simulink model "Simulation"  (R2018b)
settings: Solver=VariableStepAuto  StartTime=0.0  StopTime=tmax  RelTol=1e-3
values from neighbouring files (symbols this model uses):
  BPden = [1 alpha]    [RunSimulation.m]
  BPnum = [0.3 alpha]    [RunSimulation.m]
  c = 250    [RunSimulation.m]
  Fb = -1*m    (= -90000)    [RunSimulation.m]
  l = 18    [RunSimulation.m]
  m = 90000    [RunSimulation.m]    (also in TractionCurve.m = 22500)
  p0 = 0    [RunSimulation.m]
  Pres = 0/1000*[5.7/771 0 1.6]    [RunSimulation.m]
  RBD = 5    [RunSimulation.m]
  tl = .1    (= 0.1)    [RunSimulation.m]
  v0 = 100/3.6    (= 27.7777777778)    [RunSimulation.m]
  VBD = 3.5    [RunSimulation.m]
(part 1 of 3)
settings Model: Creator=raphael  LastModifiedBy=raphael

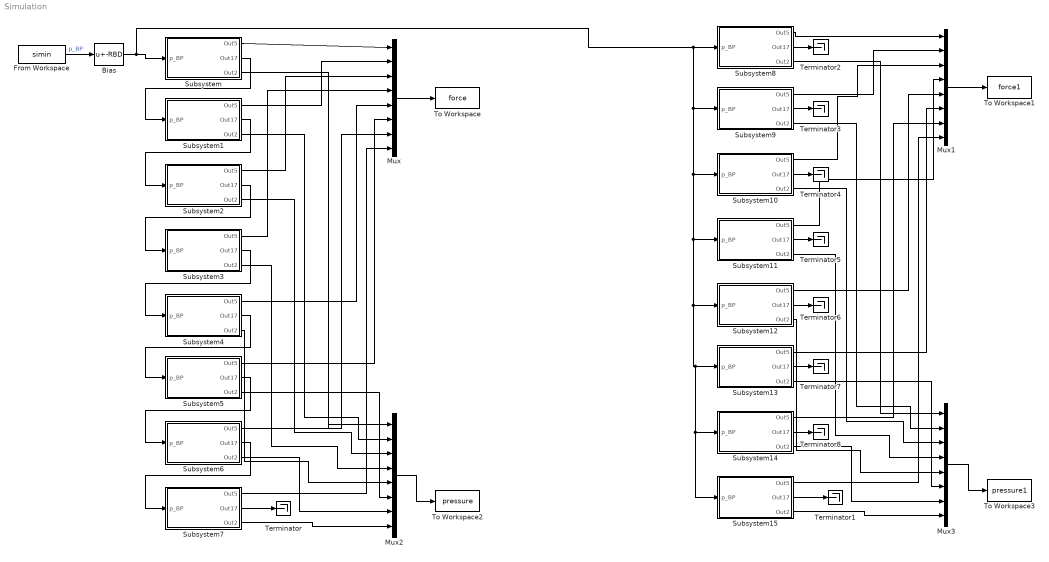
== system Simulation ==
  Bias : Bias  Bias=-RBD
  From Workspace : FromWorkspace  VariableName=simin  SampleTime=0
  Mux{,1..3} (4 alike) : Mux  Inputs=8
  Subsystem : Subsystem
  Subsystem1 : Subsystem
  Subsystem10 : Subsystem
  Subsystem11 : Subsystem
  Subsystem12 : Subsystem
  Subsystem13 : Subsystem
  Subsystem14 : Subsystem
  Subsystem15 : Subsystem
  Subsystem2 : Subsystem
  Subsystem3 : Subsystem
  Subsystem4 : Subsystem
  Subsystem5 : Subsystem
  Subsystem6 : Subsystem
  Subsystem7 : Subsystem
  Subsystem8 : Subsystem
  Subsystem9 : Subsystem
  Terminator{,1..8} (9 alike) : Terminator
  To Workspace : ToWorkspace  VariableName=force  SaveFormat=Timeseries  SampleTime=-1
  To Workspace1 : ToWorkspace  VariableName=force1  SaveFormat=Timeseries  SampleTime=-1
  To Workspace2 : ToWorkspace  VariableName=pressure  SaveFormat=Timeseries  SampleTime=-1
  To Workspace3 : ToWorkspace  VariableName=pressure1  SaveFormat=Timeseries  SampleTime=-1
  wires:
  Mux/1 -> To Workspace/1
  Mux2/1 -> To Workspace2/1
  From Workspace/1 -> Bias/1  "p_BP"
  Bias/1 -> Subsystem15/1(p_BP), Subsystem14/1(p_BP), Subsystem13/1(p_BP), Subsystem12/1(p_BP), Subsystem11/1(p_BP), Subsystem10/1(p_BP), Subsystem9/1(p_BP), Subsystem8/1(p_BP), Subsystem/1(p_BP)
  Subsystem/2(Out17) -> Subsystem1/1(p_BP)
  Subsystem1/2(Out17) -> Subsystem2/1(p_BP)
  Subsystem2/2(Out17) -> Subsystem3/1(p_BP)
  Subsystem3/2(Out17) -> Subsystem4/1(p_BP)
  Subsystem4/2(Out17) -> Subsystem5/1(p_BP)
  Subsystem5/2(Out17) -> Subsystem6/1(p_BP)
  Subsystem6/2(Out17) -> Subsystem7/1(p_BP)
  Subsystem7/2(Out17) -> Terminator/1
  Subsystem/1(Out5) -> Mux/1
  Subsystem1/1(Out5) -> Mux/2
  Subsystem2/1(Out5) -> Mux/3
  Subsystem3/1(Out5) -> Mux/4
  Subsystem4/1(Out5) -> Mux/5
  Subsystem5/1(Out5) -> Mux/6
  Subsystem6/1(Out5) -> Mux/7
  Subsystem7/1(Out5) -> Mux/8
  Subsystem1/3(Out2) -> Mux2/2
  Subsystem2/3(Out2) -> Mux2/3
  Subsystem3/3(Out2) -> Mux2/4
  Subsystem4/3(Out2) -> Mux2/5
  Subsystem/3(Out2) -> Mux2/1
  Subsystem5/3(Out2) -> Mux2/6
  Subsystem6/3(Out2) -> Mux2/7
  Subsystem7/3(Out2) -> Mux2/8
  Subsystem15/2(Out17) -> Terminator1/1
  Subsystem11/1(Out5) -> Mux1/4
  Subsystem8/3(Out2) -> Mux3/1
  Subsystem12/1(Out5) -> Mux1/5
  Subsystem8/1(Out5) -> Mux1/1
  Subsystem10/1(Out5) -> Mux1/3
  Subsystem9/3(Out2) -> Mux3/2
  Subsystem14/3(Out2) -> Mux3/7
  Subsystem14/1(Out5) -> Mux1/7
  Mux1/1 -> To Workspace1/1
  Subsystem10/3(Out2) -> Mux3/3
  Subsystem9/1(Out5) -> Mux1/2
  Subsystem12/3(Out2) -> Mux3/5
  Subsystem13/1(Out5) -> Mux1/6
  Mux3/1 -> To Workspace3/1
  Subsystem15/3(Out2) -> Mux3/8
  Subsystem13/3(Out2) -> Mux3/6
  Subsystem11/3(Out2) -> Mux3/4
  Subsystem15/1(Out5) -> Mux1/8
  Subsystem8/2(Out17) -> Terminator2/1
  Subsystem9/2(Out17) -> Terminator3/1
  Subsystem10/2(Out17) -> Terminator4/1
  Subsystem11/2(Out17) -> Terminator5/1
  Subsystem12/2(Out17) -> Terminator6/1
  Subsystem13/2(Out17) -> Terminator7/1
  Subsystem14/2(Out17) -> Terminator8/1

== system Simulation/Subsystem ==
  p_BP : Inport
  Mux : Mux  Inputs=5
  Mux2 : Mux  Inputs=5
  Wagon model : Subsystem
  Wagon model1 : Subsystem
  Wagon model2 : Subsystem
  Wagon model3 : Subsystem
  Wagon model4 : Subsystem
  Out5 : Outport
  Out17 : Outport  Port=2
  Out2 : Outport  Port=3
  wires:
  Wagon model3/2(p_BP_out) -> Mux2/4, Wagon model4/1(p_BP)
  Mux/1 -> Out5/1  "F_vec"
  Wagon model1/2(p_BP_out) -> Mux2/2, Wagon model2/1(p_BP)
  Wagon model4/2(p_BP_out) -> Out17/1, Mux2/5  "p_BP_out"
  Wagon model4/1(Fres) -> Mux/5
  Wagon model2/2(p_BP_out) -> Wagon model3/1(p_BP), Mux2/3
  Wagon model/2(p_BP_out) -> Mux2/1, Wagon model1/1(p_BP)
  Wagon model3/1(Fres) -> Mux/4
  Wagon model2/1(Fres) -> Mux/3
  Wagon model1/1(Fres) -> Mux/2
  Wagon model/1(Fres) -> Mux/1
  Mux2/1 -> Out2/1  "BP_vec"
  p_BP/1 -> Wagon model/1(p_BP)

== system Simulation/Subsystem1 ==
  p_BP : Inport
  Mux : Mux  Inputs=5
  Mux2 : Mux  Inputs=5
  Wagon model : Subsystem
  Wagon model1 : Subsystem
  Wagon model2 : Subsystem
  Wagon model3 : Subsystem
  Wagon model4 : Subsystem
  Out5 : Outport
  Out17 : Outport  Port=2
  Out2 : Outport  Port=3
  wires:
  Wagon model3/2(p_BP_out) -> Mux2/4, Wagon model4/1(p_BP)
  Mux/1 -> Out5/1  "F_vec"
  Wagon model1/2(p_BP_out) -> Mux2/2, Wagon model2/1(p_BP)
  Wagon model4/2(p_BP_out) -> Out17/1, Mux2/5  "p_BP_out"
  Wagon model4/1(Fres) -> Mux/5
  Wagon model2/2(p_BP_out) -> Wagon model3/1(p_BP), Mux2/3
  Wagon model/2(p_BP_out) -> Mux2/1, Wagon model1/1(p_BP)
  Wagon model3/1(Fres) -> Mux/4
  Wagon model2/1(Fres) -> Mux/3
  Wagon model1/1(Fres) -> Mux/2
  Wagon model/1(Fres) -> Mux/1
  Mux2/1 -> Out2/1  "BP_vec"
  p_BP/1 -> Wagon model/1(p_BP)

== system Simulation/Subsystem10 ==
  p_BP : Inport
  Mux : Mux  Inputs=5
  Mux2 : Mux  Inputs=5
  Wagon model : Subsystem
  Wagon model1 : Subsystem
  Wagon model2 : Subsystem
  Wagon model3 : Subsystem
  Wagon model4 : Subsystem
  Out5 : Outport
  Out17 : Outport  Port=2
  Out2 : Outport  Port=3
  wires:
  Wagon model3/2(p_BP_out) -> Mux2/4, Wagon model4/1(p_BP)
  Mux/1 -> Out5/1  "F_vec"
  Wagon model1/2(p_BP_out) -> Mux2/2, Wagon model2/1(p_BP)
  Wagon model4/2(p_BP_out) -> Out17/1, Mux2/5  "p_BP_out"
  Wagon model4/1(Fres) -> Mux/5
  Wagon model2/2(p_BP_out) -> Wagon model3/1(p_BP), Mux2/3
  Wagon model/2(p_BP_out) -> Mux2/1, Wagon model1/1(p_BP)
  Wagon model3/1(Fres) -> Mux/4
  Wagon model2/1(Fres) -> Mux/3
  Wagon model1/1(Fres) -> Mux/2
  Wagon model/1(Fres) -> Mux/1
  Mux2/1 -> Out2/1  "BP_vec"
  p_BP/1 -> Wagon model/1(p_BP)

== system Simulation/Subsystem11 ==
  p_BP : Inport
  Mux : Mux  Inputs=5
  Mux2 : Mux  Inputs=5
  Wagon model : Subsystem
  Wagon model1 : Subsystem
  Wagon model2 : Subsystem
  Wagon model3 : Subsystem
  Wagon model4 : Subsystem
  Out5 : Outport
  Out17 : Outport  Port=2
  Out2 : Outport  Port=3
  wires:
  Wagon model3/2(p_BP_out) -> Mux2/4, Wagon model4/1(p_BP)
  Mux/1 -> Out5/1  "F_vec"
  Wagon model1/2(p_BP_out) -> Mux2/2, Wagon model2/1(p_BP)
  Wagon model4/2(p_BP_out) -> Out17/1, Mux2/5  "p_BP_out"
  Wagon model4/1(Fres) -> Mux/5
  Wagon model2/2(p_BP_out) -> Wagon model3/1(p_BP), Mux2/3
  Wagon model/2(p_BP_out) -> Mux2/1, Wagon model1/1(p_BP)
  Wagon model3/1(Fres) -> Mux/4
  Wagon model2/1(Fres) -> Mux/3
  Wagon model1/1(Fres) -> Mux/2
  Wagon model/1(Fres) -> Mux/1
  Mux2/1 -> Out2/1  "BP_vec"
  p_BP/1 -> Wagon model/1(p_BP)

== system Simulation/Subsystem12 ==
  p_BP : Inport
  Mux : Mux  Inputs=5
  Mux2 : Mux  Inputs=5
  Wagon model : Subsystem
  Wagon model1 : Subsystem
  Wagon model2 : Subsystem
  Wagon model3 : Subsystem
  Wagon model4 : Subsystem
  Out5 : Outport
  Out17 : Outport  Port=2
  Out2 : Outport  Port=3
  wires:
  Wagon model3/2(p_BP_out) -> Mux2/4, Wagon model4/1(p_BP)
  Mux/1 -> Out5/1  "F_vec"
  Wagon model1/2(p_BP_out) -> Mux2/2, Wagon model2/1(p_BP)
  Wagon model4/2(p_BP_out) -> Out17/1, Mux2/5  "p_BP_out"
  Wagon model4/1(Fres) -> Mux/5
  Wagon model2/2(p_BP_out) -> Wagon model3/1(p_BP), Mux2/3
  Wagon model/2(p_BP_out) -> Mux2/1, Wagon model1/1(p_BP)
  Wagon model3/1(Fres) -> Mux/4
  Wagon model2/1(Fres) -> Mux/3
  Wagon model1/1(Fres) -> Mux/2
  Wagon model/1(Fres) -> Mux/1
  Mux2/1 -> Out2/1  "BP_vec"
  p_BP/1 -> Wagon model/1(p_BP)

== system Simulation/Subsystem13 ==
  p_BP : Inport
  Mux : Mux  Inputs=5
  Mux2 : Mux  Inputs=5
  Wagon model : Subsystem
  Wagon model1 : Subsystem
  Wagon model2 : Subsystem
  Wagon model3 : Subsystem
  Wagon model4 : Subsystem
  Out5 : Outport
  Out17 : Outport  Port=2
  Out2 : Outport  Port=3
  wires:
  Wagon model3/2(p_BP_out) -> Mux2/4, Wagon model4/1(p_BP)
  Mux/1 -> Out5/1  "F_vec"
  Wagon model1/2(p_BP_out) -> Mux2/2, Wagon model2/1(p_BP)
  Wagon model4/2(p_BP_out) -> Out17/1, Mux2/5  "p_BP_out"
  Wagon model4/1(Fres) -> Mux/5
  Wagon model2/2(p_BP_out) -> Wagon model3/1(p_BP), Mux2/3
  Wagon model/2(p_BP_out) -> Mux2/1, Wagon model1/1(p_BP)
  Wagon model3/1(Fres) -> Mux/4
  Wagon model2/1(Fres) -> Mux/3
  Wagon model1/1(Fres) -> Mux/2
  Wagon model/1(Fres) -> Mux/1
  Mux2/1 -> Out2/1  "BP_vec"
  p_BP/1 -> Wagon model/1(p_BP)

== system Simulation/Subsystem14 ==
  p_BP : Inport
  Mux : Mux  Inputs=5
  Mux2 : Mux  Inputs=5
  Wagon model : Subsystem
  Wagon model1 : Subsystem
  Wagon model2 : Subsystem
  Wagon model3 : Subsystem
  Wagon model4 : Subsystem
  Out5 : Outport
  Out17 : Outport  Port=2
  Out2 : Outport  Port=3
  wires:
  Wagon model3/2(p_BP_out) -> Mux2/4, Wagon model4/1(p_BP)
  Mux/1 -> Out5/1  "F_vec"
  Wagon model1/2(p_BP_out) -> Mux2/2, Wagon model2/1(p_BP)
  Wagon model4/2(p_BP_out) -> Out17/1, Mux2/5  "p_BP_out"
  Wagon model4/1(Fres) -> Mux/5
  Wagon model2/2(p_BP_out) -> Wagon model3/1(p_BP), Mux2/3
  Wagon model/2(p_BP_out) -> Mux2/1, Wagon model1/1(p_BP)
  Wagon model3/1(Fres) -> Mux/4
  Wagon model2/1(Fres) -> Mux/3
  Wagon model1/1(Fres) -> Mux/2
  Wagon model/1(Fres) -> Mux/1
  Mux2/1 -> Out2/1  "BP_vec"
  p_BP/1 -> Wagon model/1(p_BP)

== system Simulation/Subsystem15 ==
  p_BP : Inport
  Mux : Mux  Inputs=5
  Mux2 : Mux  Inputs=5
  Wagon model : Subsystem
  Wagon model1 : Subsystem
  Wagon model2 : Subsystem
  Wagon model3 : Subsystem
  Wagon model4 : Subsystem
  Out5 : Outport
  Out17 : Outport  Port=2
  Out2 : Outport  Port=3
  wires:
  Wagon model3/2(p_BP_out) -> Mux2/4, Wagon model4/1(p_BP)
  Mux/1 -> Out5/1  "F_vec"
  Wagon model1/2(p_BP_out) -> Mux2/2, Wagon model2/1(p_BP)
  Wagon model4/2(p_BP_out) -> Out17/1, Mux2/5  "p_BP_out"
  Wagon model4/1(Fres) -> Mux/5
  Wagon model2/2(p_BP_out) -> Wagon model3/1(p_BP), Mux2/3
  Wagon model/2(p_BP_out) -> Mux2/1, Wagon model1/1(p_BP)
  Wagon model3/1(Fres) -> Mux/4
  Wagon model2/1(Fres) -> Mux/3
  Wagon model1/1(Fres) -> Mux/2
  Wagon model/1(Fres) -> Mux/1
  Mux2/1 -> Out2/1  "BP_vec"
  p_BP/1 -> Wagon model/1(p_BP)

== system Simulation/Subsystem2 ==
  p_BP : Inport
  Mux : Mux  Inputs=5
  Mux2 : Mux  Inputs=5
  Wagon model : Subsystem
  Wagon model1 : Subsystem
  Wagon model2 : Subsystem
  Wagon model3 : Subsystem
  Wagon model4 : Subsystem
  Out5 : Outport
  Out17 : Outport  Port=2
  Out2 : Outport  Port=3
  wires:
  Wagon model3/2(p_BP_out) -> Mux2/4, Wagon model4/1(p_BP)
  Mux/1 -> Out5/1  "F_vec"
  Wagon model1/2(p_BP_out) -> Mux2/2, Wagon model2/1(p_BP)
  Wagon model4/2(p_BP_out) -> Out17/1, Mux2/5  "p_BP_out"
  Wagon model4/1(Fres) -> Mux/5
  Wagon model2/2(p_BP_out) -> Wagon model3/1(p_BP), Mux2/3
  Wagon model/2(p_BP_out) -> Mux2/1, Wagon model1/1(p_BP)
  Wagon model3/1(Fres) -> Mux/4
  Wagon model2/1(Fres) -> Mux/3
  Wagon model1/1(Fres) -> Mux/2
  Wagon model/1(Fres) -> Mux/1
  Mux2/1 -> Out2/1  "BP_vec"
  p_BP/1 -> Wagon model/1(p_BP)

== system Simulation/Subsystem3 ==
  p_BP : Inport
  Mux : Mux  Inputs=5
  Mux2 : Mux  Inputs=5
  Wagon model : Subsystem
  Wagon model1 : Subsystem
  Wagon model2 : Subsystem
  Wagon model3 : Subsystem
  Wagon model4 : Subsystem
  Out5 : Outport
  Out17 : Outport  Port=2
  Out2 : Outport  Port=3
  wires:
  Wagon model3/2(p_BP_out) -> Mux2/4, Wagon model4/1(p_BP)
  Mux/1 -> Out5/1  "F_vec"
  Wagon model1/2(p_BP_out) -> Mux2/2, Wagon model2/1(p_BP)
  Wagon model4/2(p_BP_out) -> Out17/1, Mux2/5  "p_BP_out"
  Wagon model4/1(Fres) -> Mux/5
  Wagon model2/2(p_BP_out) -> Wagon model3/1(p_BP), Mux2/3
  Wagon model/2(p_BP_out) -> Mux2/1, Wagon model1/1(p_BP)
  Wagon model3/1(Fres) -> Mux/4
  Wagon model2/1(Fres) -> Mux/3
  Wagon model1/1(Fres) -> Mux/2
  Wagon model/1(Fres) -> Mux/1
  Mux2/1 -> Out2/1  "BP_vec"
  p_BP/1 -> Wagon model/1(p_BP)

== system Simulation/Subsystem4 ==
  p_BP : Inport
  Mux : Mux  Inputs=5
  Mux2 : Mux  Inputs=5
  Wagon model : Subsystem
  Wagon model1 : Subsystem
  Wagon model2 : Subsystem
  Wagon model3 : Subsystem
  Wagon model4 : Subsystem
  Out5 : Outport
  Out17 : Outport  Port=2
  Out2 : Outport  Port=3
  wires:
  Wagon model3/2(p_BP_out) -> Mux2/4, Wagon model4/1(p_BP)
  Mux/1 -> Out5/1  "F_vec"
  Wagon model1/2(p_BP_out) -> Mux2/2, Wagon model2/1(p_BP)
  Wagon model4/2(p_BP_out) -> Out17/1, Mux2/5  "p_BP_out"
  Wagon model4/1(Fres) -> Mux/5
  Wagon model2/2(p_BP_out) -> Wagon model3/1(p_BP), Mux2/3
  Wagon model/2(p_BP_out) -> Mux2/1, Wagon model1/1(p_BP)
  Wagon model3/1(Fres) -> Mux/4
  Wagon model2/1(Fres) -> Mux/3
  Wagon model1/1(Fres) -> Mux/2
  Wagon model/1(Fres) -> Mux/1
  Mux2/1 -> Out2/1  "BP_vec"
  p_BP/1 -> Wagon model/1(p_BP)

== system Simulation/Subsystem5 ==
  p_BP : Inport
  Mux : Mux  Inputs=5
  Mux2 : Mux  Inputs=5
  Wagon model : Subsystem
  Wagon model1 : Subsystem
  Wagon model2 : Subsystem
  Wagon model3 : Subsystem
  Wagon model4 : Subsystem
  Out5 : Outport
  Out17 : Outport  Port=2
  Out2 : Outport  Port=3
  wires:
  Wagon model3/2(p_BP_out) -> Mux2/4, Wagon model4/1(p_BP)
  Mux/1 -> Out5/1  "F_vec"
  Wagon model1/2(p_BP_out) -> Mux2/2, Wagon model2/1(p_BP)
  Wagon model4/2(p_BP_out) -> Out17/1, Mux2/5  "p_BP_out"
  Wagon model4/1(Fres) -> Mux/5
  Wagon model2/2(p_BP_out) -> Wagon model3/1(p_BP), Mux2/3
  Wagon model/2(p_BP_out) -> Mux2/1, Wagon model1/1(p_BP)
  Wagon model3/1(Fres) -> Mux/4
  Wagon model2/1(Fres) -> Mux/3
  Wagon model1/1(Fres) -> Mux/2
  Wagon model/1(Fres) -> Mux/1
  Mux2/1 -> Out2/1  "BP_vec"
  p_BP/1 -> Wagon model/1(p_BP)

== system Simulation/Subsystem6 ==
  p_BP : Inport
  Mux : Mux  Inputs=5
  Mux2 : Mux  Inputs=5
  Wagon model : Subsystem
  Wagon model1 : Subsystem
  Wagon model2 : Subsystem
  Wagon model3 : Subsystem
  Wagon model4 : Subsystem
  Out5 : Outport
  Out17 : Outport  Port=2
  Out2 : Outport  Port=3
  wires:
  Wagon model3/2(p_BP_out) -> Mux2/4, Wagon model4/1(p_BP)
  Mux/1 -> Out5/1  "F_vec"
  Wagon model1/2(p_BP_out) -> Mux2/2, Wagon model2/1(p_BP)
  Wagon model4/2(p_BP_out) -> Out17/1, Mux2/5  "p_BP_out"
  Wagon model4/1(Fres) -> Mux/5
  Wagon model2/2(p_BP_out) -> Wagon model3/1(p_BP), Mux2/3
  Wagon model/2(p_BP_out) -> Mux2/1, Wagon model1/1(p_BP)
  Wagon model3/1(Fres) -> Mux/4
  Wagon model2/1(Fres) -> Mux/3
  Wagon model1/1(Fres) -> Mux/2
  Wagon model/1(Fres) -> Mux/1
  Mux2/1 -> Out2/1  "BP_vec"
  p_BP/1 -> Wagon model/1(p_BP)

== system Simulation/Subsystem7 ==
  p_BP : Inport
  Mux : Mux  Inputs=5
  Mux2 : Mux  Inputs=5
  Wagon model : Subsystem
  Wagon model1 : Subsystem
  Wagon model2 : Subsystem
  Wagon model3 : Subsystem
  Wagon model4 : Subsystem
  Out5 : Outport
  Out17 : Outport  Port=2
  Out2 : Outport  Port=3
  wires:
  Wagon model3/2(p_BP_out) -> Mux2/4, Wagon model4/1(p_BP)
  Mux/1 -> Out5/1  "F_vec"
  Wagon model1/2(p_BP_out) -> Mux2/2, Wagon model2/1(p_BP)
  Wagon model4/2(p_BP_out) -> Out17/1, Mux2/5  "p_BP_out"
  Wagon model4/1(Fres) -> Mux/5
  Wagon model2/2(p_BP_out) -> Wagon model3/1(p_BP), Mux2/3
  Wagon model/2(p_BP_out) -> Mux2/1, Wagon model1/1(p_BP)
  Wagon model3/1(Fres) -> Mux/4
  Wagon model2/1(Fres) -> Mux/3
  Wagon model1/1(Fres) -> Mux/2
  Wagon model/1(Fres) -> Mux/1
  Mux2/1 -> Out2/1  "BP_vec"
  p_BP/1 -> Wagon model/1(p_BP)

== system Simulation/Subsystem8 ==
  p_BP : Inport
  Mux : Mux  Inputs=5
  Mux2 : Mux  Inputs=5
  Wagon model : Subsystem
  Wagon model1 : Subsystem
  Wagon model2 : Subsystem
  Wagon model3 : Subsystem
  Wagon model4 : Subsystem
  Out5 : Outport
  Out17 : Outport  Port=2
  Out2 : Outport  Port=3
  wires:
  Wagon model3/2(p_BP_out) -> Mux2/4, Wagon model4/1(p_BP)
  Mux/1 -> Out5/1  "F_vec"
  Wagon model1/2(p_BP_out) -> Mux2/2, Wagon model2/1(p_BP)
  Wagon model4/2(p_BP_out) -> Out17/1, Mux2/5  "p_BP_out"
  Wagon model4/1(Fres) -> Mux/5
  Wagon model2/2(p_BP_out) -> Wagon model3/1(p_BP), Mux2/3
  Wagon model/2(p_BP_out) -> Mux2/1, Wagon model1/1(p_BP)
  Wagon model3/1(Fres) -> Mux/4
  Wagon model2/1(Fres) -> Mux/3
  Wagon model1/1(Fres) -> Mux/2
  Wagon model/1(Fres) -> Mux/1
  Mux2/1 -> Out2/1  "BP_vec"
  p_BP/1 -> Wagon model/1(p_BP)

== system Simulation/Subsystem9 ==
  p_BP : Inport
  Mux : Mux  Inputs=5
  Mux2 : Mux  Inputs=5
  Wagon model : Subsystem
  Wagon model1 : Subsystem
  Wagon model2 : Subsystem
  Wagon model3 : Subsystem
  Wagon model4 : Subsystem
  Out5 : Outport
  Out17 : Outport  Port=2
  Out2 : Outport  Port=3
  wires:
  Wagon model3/2(p_BP_out) -> Mux2/4, Wagon model4/1(p_BP)
  Mux/1 -> Out5/1  "F_vec"
  Wagon model1/2(p_BP_out) -> Mux2/2, Wagon model2/1(p_BP)
  Wagon model4/2(p_BP_out) -> Out17/1, Mux2/5  "p_BP_out"
  Wagon model4/1(Fres) -> Mux/5
  Wagon model2/2(p_BP_out) -> Wagon model3/1(p_BP), Mux2/3
  Wagon model/2(p_BP_out) -> Mux2/1, Wagon model1/1(p_BP)
  Wagon model3/1(Fres) -> Mux/4
  Wagon model2/1(Fres) -> Mux/3
  Wagon model1/1(Fres) -> Mux/2
  Wagon model/1(Fres) -> Mux/1
  Mux2/1 -> Out2/1  "BP_vec"
  p_BP/1 -> Wagon model/1(p_BP)

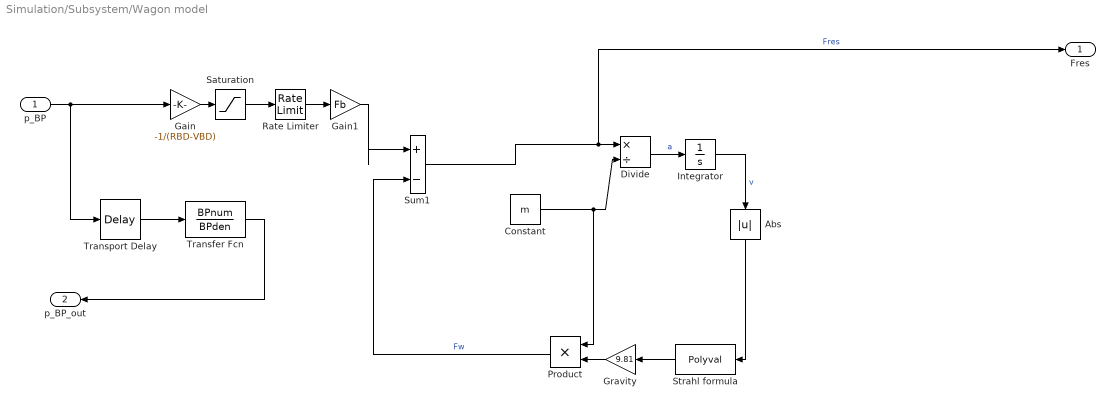
== system Simulation/Subsystem/Wagon model ==
  p_BP : Inport
  Abs : Abs
  Constant : Constant  Value=m
  Divide : Product  Inputs=*/
  Gain : Gain  Gain=-1/(RBD-VBD)
  Gain1 : Gain  Gain=Fb
  Gravity : Gain  Gain=9.81
  Integrator : Integrator  InitialCondition=v0
  Product : Product
  Rate Limiter : RateLimiter  RisingSlewLimit=1/tf  FallingSlewLimit=-1/tl  SampleTimeMode=inherited
  Saturation : Saturate  UpperLimit=1  LowerLimit=0
  Strahl formula : Polyval  Coefs=Pres
  Sum1 : Sum  Inputs=|+-
  Transfer Fcn : TransferFcn  Numerator=BPnum  Denominator=BPden
  Transport Delay : TransportDelay  DelayTime=l/c  InitialOutput=p0
  Fres : Outport
  p_BP_out : Outport  Port=2
  wires:
  Sum1/1 -> Fres/1, Divide/1  "Fres"
  Strahl formula/1 -> Gravity/1
  Abs/1 -> Strahl formula/1
  Gravity/1 -> Product/2
  Product/1 -> Sum1/2  "Fw"
  Integrator/1 -> Abs/1  "v"
  Constant/1 -> Product/1, Divide/2
  Divide/1 -> Integrator/1  "a"
  p_BP/1 -> Gain/1, Transport Delay/1
  Gain/1 -> Saturation/1
  Gain1/1 -> Sum1/1
  Saturation/1 -> Rate Limiter/1
  Rate Limiter/1 -> Gain1/1
  Transfer Fcn/1 -> p_BP_out/1
  Transport Delay/1 -> Transfer Fcn/1

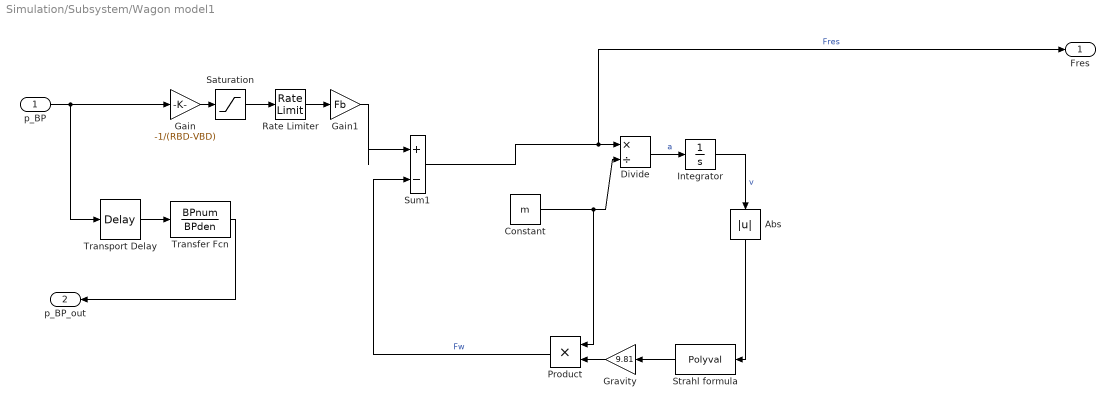
== system Simulation/Subsystem/Wagon model1 ==
  p_BP : Inport
  Abs : Abs
  Constant : Constant  Value=m
  Divide : Product  Inputs=*/
  Gain : Gain  Gain=-1/(RBD-VBD)
  Gain1 : Gain  Gain=Fb
  Gravity : Gain  Gain=9.81
  Integrator : Integrator  InitialCondition=v0
  Product : Product
  Rate Limiter : RateLimiter  RisingSlewLimit=1/tf  FallingSlewLimit=-1/tl  SampleTimeMode=inherited
  Saturation : Saturate  UpperLimit=1  LowerLimit=0
  Strahl formula : Polyval  Coefs=Pres
  Sum1 : Sum  Inputs=|+-
  Transfer Fcn : TransferFcn  Numerator=BPnum  Denominator=BPden
  Transport Delay : TransportDelay  DelayTime=l/c  InitialOutput=p0
  Fres : Outport
  p_BP_out : Outport  Port=2
  wires:
  Sum1/1 -> Fres/1, Divide/1  "Fres"
  Strahl formula/1 -> Gravity/1
  Abs/1 -> Strahl formula/1
  Gravity/1 -> Product/2
  Product/1 -> Sum1/2  "Fw"
  Integrator/1 -> Abs/1  "v"
  Constant/1 -> Product/1, Divide/2
  Divide/1 -> Integrator/1  "a"
  p_BP/1 -> Gain/1, Transport Delay/1
  Gain/1 -> Saturation/1
  Gain1/1 -> Sum1/1
  Saturation/1 -> Rate Limiter/1
  Rate Limiter/1 -> Gain1/1
  Transport Delay/1 -> Transfer Fcn/1
  Transfer Fcn/1 -> p_BP_out/1

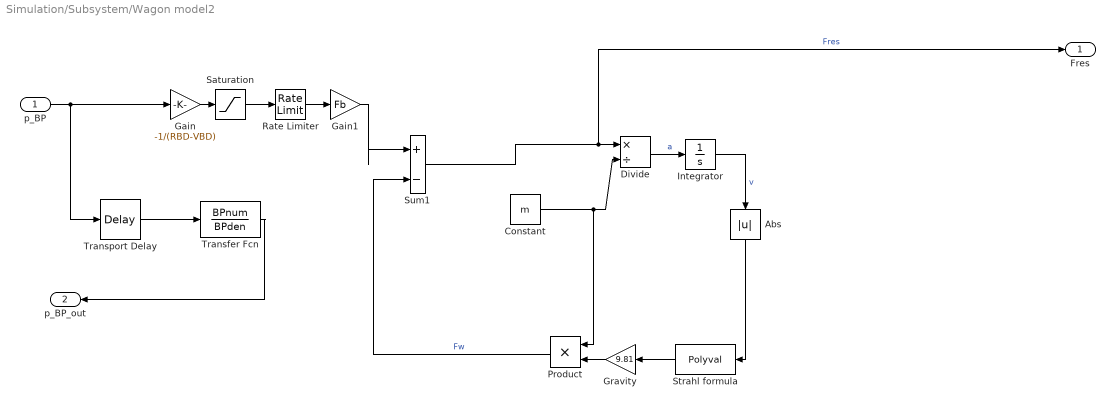
== system Simulation/Subsystem/Wagon model2 ==
  p_BP : Inport
  Abs : Abs
  Constant : Constant  Value=m
  Divide : Product  Inputs=*/
  Gain : Gain  Gain=-1/(RBD-VBD)
  Gain1 : Gain  Gain=Fb
  Gravity : Gain  Gain=9.81
  Integrator : Integrator  InitialCondition=v0
  Product : Product
  Rate Limiter : RateLimiter  RisingSlewLimit=1/tf  FallingSlewLimit=-1/tl  SampleTimeMode=inherited
  Saturation : Saturate  UpperLimit=1  LowerLimit=0
  Strahl formula : Polyval  Coefs=Pres
  Sum1 : Sum  Inputs=|+-
  Transfer Fcn : TransferFcn  Numerator=BPnum  Denominator=BPden
  Transport Delay : TransportDelay  DelayTime=l/c  InitialOutput=p0
  Fres : Outport
  p_BP_out : Outport  Port=2
  wires:
  Sum1/1 -> Fres/1, Divide/1  "Fres"
  Strahl formula/1 -> Gravity/1
  Abs/1 -> Strahl formula/1
  Gravity/1 -> Product/2
  Product/1 -> Sum1/2  "Fw"
  Constant/1 -> Product/1, Divide/2
  Divide/1 -> Integrator/1  "a"
  p_BP/1 -> Gain/1, Transport Delay/1
  Gain/1 -> Saturation/1
  Gain1/1 -> Sum1/1
  Saturation/1 -> Rate Limiter/1
  Rate Limiter/1 -> Gain1/1
  Transport Delay/1 -> Transfer Fcn/1
  Transfer Fcn/1 -> p_BP_out/1
  Integrator/1 -> Abs/1  "v"

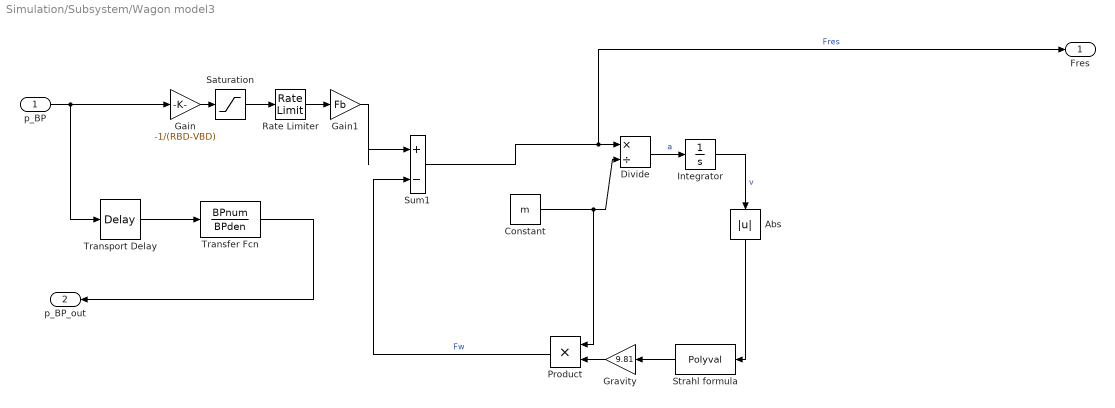
== system Simulation/Subsystem/Wagon model3 ==
  p_BP : Inport
  Abs : Abs
  Constant : Constant  Value=m
  Divide : Product  Inputs=*/
  Gain : Gain  Gain=-1/(RBD-VBD)
  Gain1 : Gain  Gain=Fb
  Gravity : Gain  Gain=9.81
  Integrator : Integrator  InitialCondition=v0
  Product : Product
  Rate Limiter : RateLimiter  RisingSlewLimit=1/tf  FallingSlewLimit=-1/tl  SampleTimeMode=inherited
  Saturation : Saturate  UpperLimit=1  LowerLimit=0
  Strahl formula : Polyval  Coefs=Pres
  Sum1 : Sum  Inputs=|+-
  Transfer Fcn : TransferFcn  Numerator=BPnum  Denominator=BPden
  Transport Delay : TransportDelay  DelayTime=l/c  InitialOutput=p0
  Fres : Outport
  p_BP_out : Outport  Port=2
  wires:
  Sum1/1 -> Fres/1, Divide/1  "Fres"
  Strahl formula/1 -> Gravity/1
  Abs/1 -> Strahl formula/1
  Gravity/1 -> Product/2
  Product/1 -> Sum1/2  "Fw"
  Constant/1 -> Product/1, Divide/2
  Divide/1 -> Integrator/1  "a"
  p_BP/1 -> Gain/1, Transport Delay/1
  Gain/1 -> Saturation/1
  Gain1/1 -> Sum1/1
  Saturation/1 -> Rate Limiter/1
  Rate Limiter/1 -> Gain1/1
  Transport Delay/1 -> Transfer Fcn/1
  Transfer Fcn/1 -> p_BP_out/1
  Integrator/1 -> Abs/1  "v"

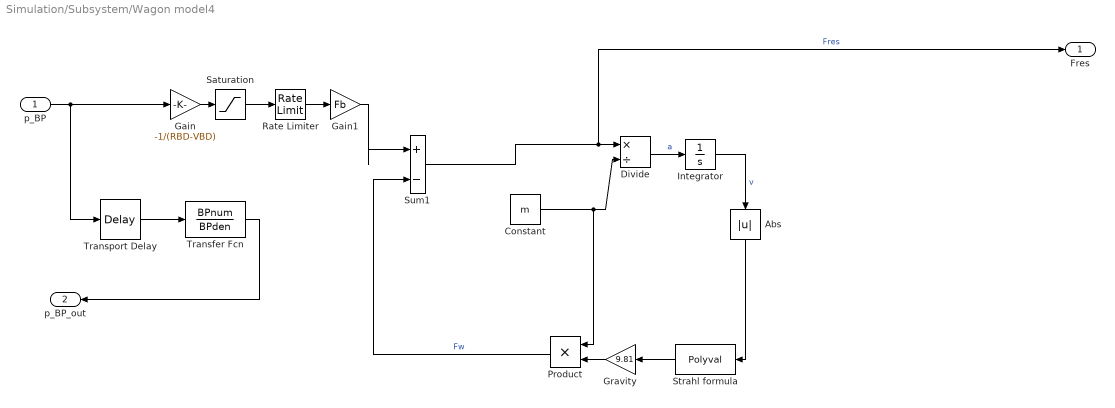
== system Simulation/Subsystem/Wagon model4 ==
  p_BP : Inport
  Abs : Abs
  Constant : Constant  Value=m
  Divide : Product  Inputs=*/
  Gain : Gain  Gain=-1/(RBD-VBD)
  Gain1 : Gain  Gain=Fb
  Gravity : Gain  Gain=9.81
  Integrator : Integrator  InitialCondition=v0
  Product : Product
  Rate Limiter : RateLimiter  RisingSlewLimit=1/tf  FallingSlewLimit=-1/tl  SampleTimeMode=inherited
  Saturation : Saturate  UpperLimit=1  LowerLimit=0
  Strahl formula : Polyval  Coefs=Pres
  Sum1 : Sum  Inputs=|+-
  Transfer Fcn : TransferFcn  Numerator=BPnum  Denominator=BPden
  Transport Delay : TransportDelay  DelayTime=l/c  InitialOutput=p0
  Fres : Outport
  p_BP_out : Outport  Port=2
  wires:
  Sum1/1 -> Fres/1, Divide/1  "Fres"
  Strahl formula/1 -> Gravity/1
  Abs/1 -> Strahl formula/1
  Gravity/1 -> Product/2
  Product/1 -> Sum1/2  "Fw"
  Integrator/1 -> Abs/1  "v"
  Constant/1 -> Product/1, Divide/2
  Divide/1 -> Integrator/1  "a"
  p_BP/1 -> Gain/1, Transport Delay/1
  Gain/1 -> Saturation/1
  Gain1/1 -> Sum1/1
  Saturation/1 -> Rate Limiter/1
  Rate Limiter/1 -> Gain1/1
  Transfer Fcn/1 -> p_BP_out/1
  Transport Delay/1 -> Transfer Fcn/1

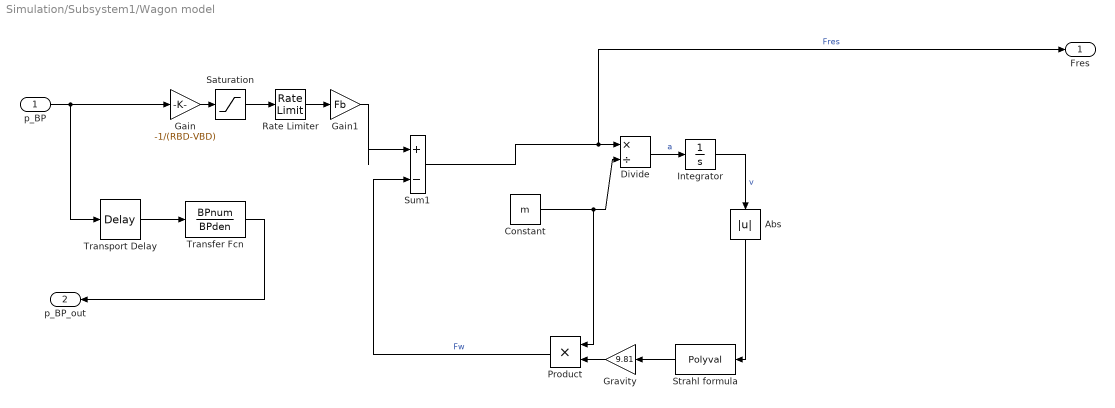
== system Simulation/Subsystem1/Wagon model ==
  p_BP : Inport
  Abs : Abs
  Constant : Constant  Value=m
  Divide : Product  Inputs=*/
  Gain : Gain  Gain=-1/(RBD-VBD)
  Gain1 : Gain  Gain=Fb
  Gravity : Gain  Gain=9.81
  Integrator : Integrator  InitialCondition=v0
  Product : Product
  Rate Limiter : RateLimiter  RisingSlewLimit=1/tf  FallingSlewLimit=-1/tl  SampleTimeMode=inherited
  Saturation : Saturate  UpperLimit=1  LowerLimit=0
  Strahl formula : Polyval  Coefs=Pres
  Sum1 : Sum  Inputs=|+-
  Transfer Fcn : TransferFcn  Numerator=BPnum  Denominator=BPden
  Transport Delay : TransportDelay  DelayTime=l/c  InitialOutput=p0
  Fres : Outport
  p_BP_out : Outport  Port=2
  wires:
  Sum1/1 -> Fres/1, Divide/1  "Fres"
  Strahl formula/1 -> Gravity/1
  Abs/1 -> Strahl formula/1
  Gravity/1 -> Product/2
  Product/1 -> Sum1/2  "Fw"
  Integrator/1 -> Abs/1  "v"
  Constant/1 -> Product/1, Divide/2
  Divide/1 -> Integrator/1  "a"
  p_BP/1 -> Gain/1, Transport Delay/1
  Gain/1 -> Saturation/1
  Gain1/1 -> Sum1/1
  Saturation/1 -> Rate Limiter/1
  Rate Limiter/1 -> Gain1/1
  Transfer Fcn/1 -> p_BP_out/1
  Transport Delay/1 -> Transfer Fcn/1

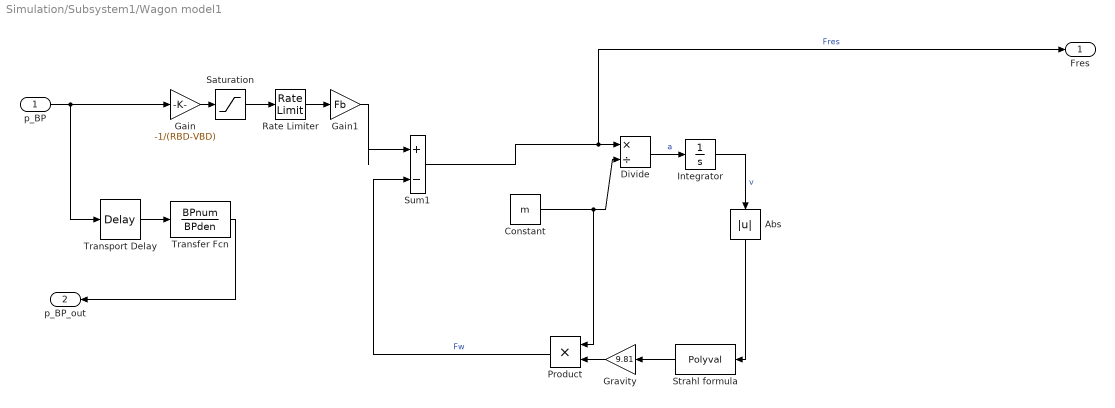
== system Simulation/Subsystem1/Wagon model1 ==
  p_BP : Inport
  Abs : Abs
  Constant : Constant  Value=m
  Divide : Product  Inputs=*/
  Gain : Gain  Gain=-1/(RBD-VBD)
  Gain1 : Gain  Gain=Fb
  Gravity : Gain  Gain=9.81
  Integrator : Integrator  InitialCondition=v0
  Product : Product
  Rate Limiter : RateLimiter  RisingSlewLimit=1/tf  FallingSlewLimit=-1/tl  SampleTimeMode=inherited
  Saturation : Saturate  UpperLimit=1  LowerLimit=0
  Strahl formula : Polyval  Coefs=Pres
  Sum1 : Sum  Inputs=|+-
  Transfer Fcn : TransferFcn  Numerator=BPnum  Denominator=BPden
  Transport Delay : TransportDelay  DelayTime=l/c  InitialOutput=p0
  Fres : Outport
  p_BP_out : Outport  Port=2
  wires:
  Sum1/1 -> Fres/1, Divide/1  "Fres"
  Strahl formula/1 -> Gravity/1
  Abs/1 -> Strahl formula/1
  Gravity/1 -> Product/2
  Product/1 -> Sum1/2  "Fw"
  Integrator/1 -> Abs/1  "v"
  Constant/1 -> Product/1, Divide/2
  Divide/1 -> Integrator/1  "a"
  p_BP/1 -> Gain/1, Transport Delay/1
  Gain/1 -> Saturation/1
  Gain1/1 -> Sum1/1
  Saturation/1 -> Rate Limiter/1
  Rate Limiter/1 -> Gain1/1
  Transport Delay/1 -> Transfer Fcn/1
  Transfer Fcn/1 -> p_BP_out/1

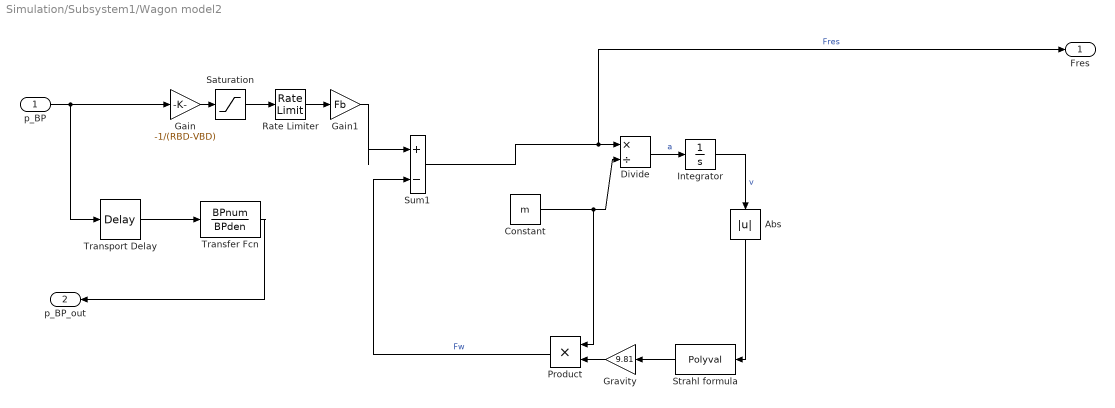
== system Simulation/Subsystem1/Wagon model2 ==
  p_BP : Inport
  Abs : Abs
  Constant : Constant  Value=m
  Divide : Product  Inputs=*/
  Gain : Gain  Gain=-1/(RBD-VBD)
  Gain1 : Gain  Gain=Fb
  Gravity : Gain  Gain=9.81
  Integrator : Integrator  InitialCondition=v0
  Product : Product
  Rate Limiter : RateLimiter  RisingSlewLimit=1/tf  FallingSlewLimit=-1/tl  SampleTimeMode=inherited
  Saturation : Saturate  UpperLimit=1  LowerLimit=0
  Strahl formula : Polyval  Coefs=Pres
  Sum1 : Sum  Inputs=|+-
  Transfer Fcn : TransferFcn  Numerator=BPnum  Denominator=BPden
  Transport Delay : TransportDelay  DelayTime=l/c  InitialOutput=p0
  Fres : Outport
  p_BP_out : Outport  Port=2
  wires:
  Sum1/1 -> Fres/1, Divide/1  "Fres"
  Strahl formula/1 -> Gravity/1
  Abs/1 -> Strahl formula/1
  Gravity/1 -> Product/2
  Product/1 -> Sum1/2  "Fw"
  Constant/1 -> Product/1, Divide/2
  Divide/1 -> Integrator/1  "a"
  p_BP/1 -> Gain/1, Transport Delay/1
  Gain/1 -> Saturation/1
  Gain1/1 -> Sum1/1
  Saturation/1 -> Rate Limiter/1
  Rate Limiter/1 -> Gain1/1
  Transport Delay/1 -> Transfer Fcn/1
  Transfer Fcn/1 -> p_BP_out/1
  Integrator/1 -> Abs/1  "v"

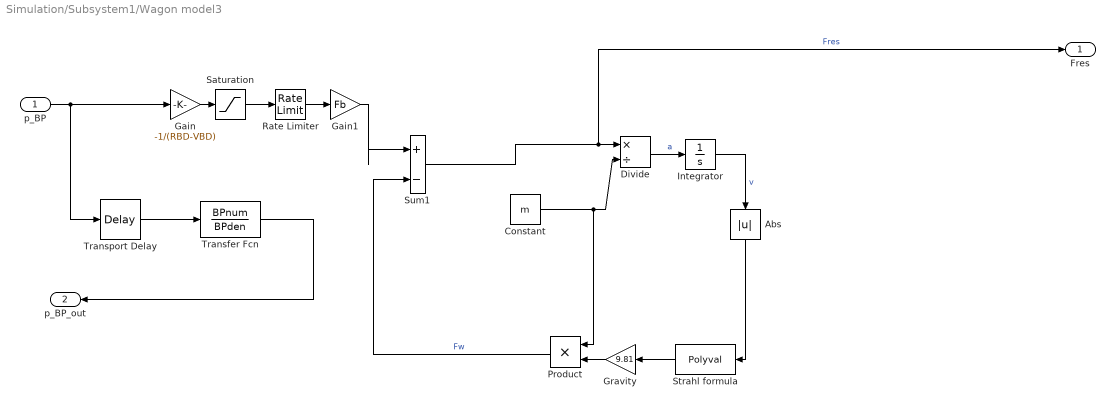
== system Simulation/Subsystem1/Wagon model3 ==
  p_BP : Inport
  Abs : Abs
  Constant : Constant  Value=m
  Divide : Product  Inputs=*/
  Gain : Gain  Gain=-1/(RBD-VBD)
  Gain1 : Gain  Gain=Fb
  Gravity : Gain  Gain=9.81
  Integrator : Integrator  InitialCondition=v0
  Product : Product
  Rate Limiter : RateLimiter  RisingSlewLimit=1/tf  FallingSlewLimit=-1/tl  SampleTimeMode=inherited
  Saturation : Saturate  UpperLimit=1  LowerLimit=0
  Strahl formula : Polyval  Coefs=Pres
  Sum1 : Sum  Inputs=|+-
  Transfer Fcn : TransferFcn  Numerator=BPnum  Denominator=BPden
  Transport Delay : TransportDelay  DelayTime=l/c  InitialOutput=p0
  Fres : Outport
  p_BP_out : Outport  Port=2
  wires:
  Sum1/1 -> Fres/1, Divide/1  "Fres"
  Strahl formula/1 -> Gravity/1
  Abs/1 -> Strahl formula/1
  Gravity/1 -> Product/2
  Product/1 -> Sum1/2  "Fw"
  Constant/1 -> Product/1, Divide/2
  Divide/1 -> Integrator/1  "a"
  p_BP/1 -> Gain/1, Transport Delay/1
  Gain/1 -> Saturation/1
  Gain1/1 -> Sum1/1
  Saturation/1 -> Rate Limiter/1
  Rate Limiter/1 -> Gain1/1
  Transport Delay/1 -> Transfer Fcn/1
  Transfer Fcn/1 -> p_BP_out/1
  Integrator/1 -> Abs/1  "v"

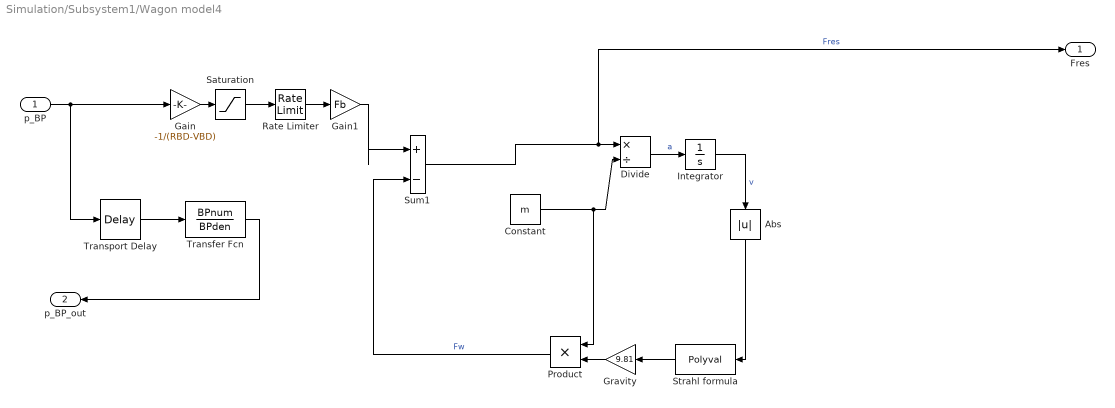
== system Simulation/Subsystem1/Wagon model4 ==
  p_BP : Inport
  Abs : Abs
  Constant : Constant  Value=m
  Divide : Product  Inputs=*/
  Gain : Gain  Gain=-1/(RBD-VBD)
  Gain1 : Gain  Gain=Fb
  Gravity : Gain  Gain=9.81
  Integrator : Integrator  InitialCondition=v0
  Product : Product
  Rate Limiter : RateLimiter  RisingSlewLimit=1/tf  FallingSlewLimit=-1/tl  SampleTimeMode=inherited
  Saturation : Saturate  UpperLimit=1  LowerLimit=0
  Strahl formula : Polyval  Coefs=Pres
  Sum1 : Sum  Inputs=|+-
  Transfer Fcn : TransferFcn  Numerator=BPnum  Denominator=BPden
  Transport Delay : TransportDelay  DelayTime=l/c  InitialOutput=p0
  Fres : Outport
  p_BP_out : Outport  Port=2
  wires:
  Sum1/1 -> Fres/1, Divide/1  "Fres"
  Strahl formula/1 -> Gravity/1
  Abs/1 -> Strahl formula/1
  Gravity/1 -> Product/2
  Product/1 -> Sum1/2  "Fw"
  Integrator/1 -> Abs/1  "v"
  Constant/1 -> Product/1, Divide/2
  Divide/1 -> Integrator/1  "a"
  p_BP/1 -> Gain/1, Transport Delay/1
  Gain/1 -> Saturation/1
  Gain1/1 -> Sum1/1
  Saturation/1 -> Rate Limiter/1
  Rate Limiter/1 -> Gain1/1
  Transfer Fcn/1 -> p_BP_out/1
  Transport Delay/1 -> Transfer Fcn/1

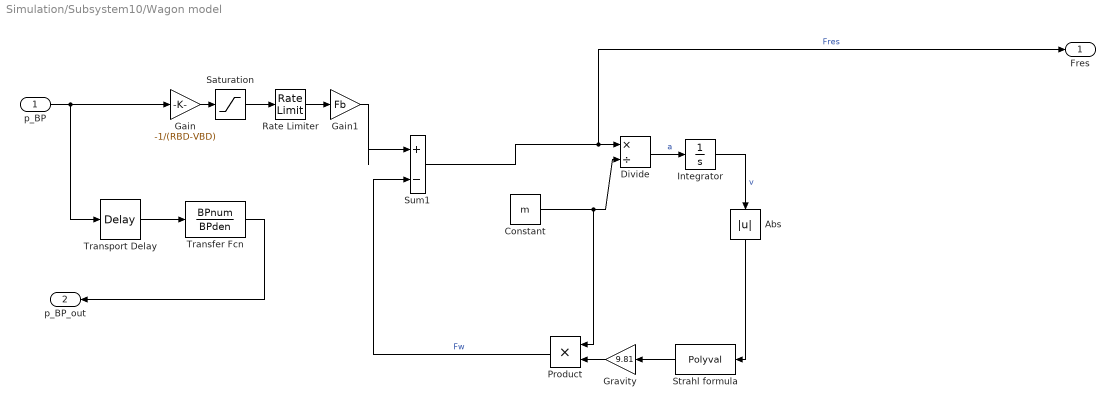
== system Simulation/Subsystem10/Wagon model ==
  p_BP : Inport
  Abs : Abs
  Constant : Constant  Value=m
  Divide : Product  Inputs=*/
  Gain : Gain  Gain=-1/(RBD-VBD)
  Gain1 : Gain  Gain=Fb
  Gravity : Gain  Gain=9.81
  Integrator : Integrator  InitialCondition=v0
  Product : Product
  Rate Limiter : RateLimiter  RisingSlewLimit=1/tf  FallingSlewLimit=-1/tl  SampleTimeMode=inherited
  Saturation : Saturate  UpperLimit=1  LowerLimit=0
  Strahl formula : Polyval  Coefs=Pres
  Sum1 : Sum  Inputs=|+-
  Transfer Fcn : TransferFcn  Numerator=BPnum  Denominator=BPden
  Transport Delay : TransportDelay  DelayTime=l/c  InitialOutput=p0
  Fres : Outport
  p_BP_out : Outport  Port=2
  wires:
  Sum1/1 -> Fres/1, Divide/1  "Fres"
  Strahl formula/1 -> Gravity/1
  Abs/1 -> Strahl formula/1
  Gravity/1 -> Product/2
  Product/1 -> Sum1/2  "Fw"
  Integrator/1 -> Abs/1  "v"
  Constant/1 -> Product/1, Divide/2
  Divide/1 -> Integrator/1  "a"
  p_BP/1 -> Gain/1, Transport Delay/1
  Gain/1 -> Saturation/1
  Gain1/1 -> Sum1/1
  Saturation/1 -> Rate Limiter/1
  Rate Limiter/1 -> Gain1/1
  Transfer Fcn/1 -> p_BP_out/1
  Transport Delay/1 -> Transfer Fcn/1

== system Simulation/Subsystem10/Wagon model1 ==
  p_BP : Inport
  Abs : Abs
  Constant : Constant  Value=m
  Divide : Product  Inputs=*/
  Gain : Gain  Gain=-1/(RBD-VBD)
  Gain1 : Gain  Gain=Fb
  Gravity : Gain  Gain=9.81
  Integrator : Integrator  InitialCondition=v0
  Product : Product
  Rate Limiter : RateLimiter  RisingSlewLimit=1/tf  FallingSlewLimit=-1/tl  SampleTimeMode=inherited
  Saturation : Saturate  UpperLimit=1  LowerLimit=0
  Strahl formula : Polyval  Coefs=Pres
  Sum1 : Sum  Inputs=|+-
  Transfer Fcn : TransferFcn  Numerator=BPnum  Denominator=BPden
  Transport Delay : TransportDelay  DelayTime=l/c  InitialOutput=p0
  Fres : Outport
  p_BP_out : Outport  Port=2
  wires:
  Sum1/1 -> Fres/1, Divide/1  "Fres"
  Strahl formula/1 -> Gravity/1
  Abs/1 -> Strahl formula/1
  Gravity/1 -> Product/2
  Product/1 -> Sum1/2  "Fw"
  Integrator/1 -> Abs/1  "v"
  Constant/1 -> Product/1, Divide/2
  Divide/1 -> Integrator/1  "a"
  p_BP/1 -> Gain/1, Transport Delay/1
  Gain/1 -> Saturation/1
  Gain1/1 -> Sum1/1
  Saturation/1 -> Rate Limiter/1
  Rate Limiter/1 -> Gain1/1
  Transport Delay/1 -> Transfer Fcn/1
  Transfer Fcn/1 -> p_BP_out/1

== system Simulation/Subsystem10/Wagon model2 ==
  p_BP : Inport
  Abs : Abs
  Constant : Constant  Value=m
  Divide : Product  Inputs=*/
  Gain : Gain  Gain=-1/(RBD-VBD)
  Gain1 : Gain  Gain=Fb
  Gravity : Gain  Gain=9.81
  Integrator : Integrator  InitialCondition=v0
  Product : Product
  Rate Limiter : RateLimiter  RisingSlewLimit=1/tf  FallingSlewLimit=-1/tl  SampleTimeMode=inherited
  Saturation : Saturate  UpperLimit=1  LowerLimit=0
  Strahl formula : Polyval  Coefs=Pres
  Sum1 : Sum  Inputs=|+-
  Transfer Fcn : TransferFcn  Numerator=BPnum  Denominator=BPden
  Transport Delay : TransportDelay  DelayTime=l/c  InitialOutput=p0
  Fres : Outport
  p_BP_out : Outport  Port=2
  wires:
  Sum1/1 -> Fres/1, Divide/1  "Fres"
  Strahl formula/1 -> Gravity/1
  Abs/1 -> Strahl formula/1
  Gravity/1 -> Product/2
  Product/1 -> Sum1/2  "Fw"
  Constant/1 -> Product/1, Divide/2
  Divide/1 -> Integrator/1  "a"
  p_BP/1 -> Gain/1, Transport Delay/1
  Gain/1 -> Saturation/1
  Gain1/1 -> Sum1/1
  Saturation/1 -> Rate Limiter/1
  Rate Limiter/1 -> Gain1/1
  Transport Delay/1 -> Transfer Fcn/1
  Transfer Fcn/1 -> p_BP_out/1
  Integrator/1 -> Abs/1  "v"

== system Simulation/Subsystem10/Wagon model3 ==
  p_BP : Inport
  Abs : Abs
  Constant : Constant  Value=m
  Divide : Product  Inputs=*/
  Gain : Gain  Gain=-1/(RBD-VBD)
  Gain1 : Gain  Gain=Fb
  Gravity : Gain  Gain=9.81
  Integrator : Integrator  InitialCondition=v0
  Product : Product
  Rate Limiter : RateLimiter  RisingSlewLimit=1/tf  FallingSlewLimit=-1/tl  SampleTimeMode=inherited
  Saturation : Saturate  UpperLimit=1  LowerLimit=0
  Strahl formula : Polyval  Coefs=Pres
  Sum1 : Sum  Inputs=|+-
  Transfer Fcn : TransferFcn  Numerator=BPnum  Denominator=BPden
  Transport Delay : TransportDelay  DelayTime=l/c  InitialOutput=p0
  Fres : Outport
  p_BP_out : Outport  Port=2
  wires:
  Sum1/1 -> Fres/1, Divide/1  "Fres"
  Strahl formula/1 -> Gravity/1
  Abs/1 -> Strahl formula/1
  Gravity/1 -> Product/2
  Product/1 -> Sum1/2  "Fw"
  Constant/1 -> Product/1, Divide/2
  Divide/1 -> Integrator/1  "a"
  p_BP/1 -> Gain/1, Transport Delay/1
  Gain/1 -> Saturation/1
  Gain1/1 -> Sum1/1
  Saturation/1 -> Rate Limiter/1
  Rate Limiter/1 -> Gain1/1
  Transport Delay/1 -> Transfer Fcn/1
  Transfer Fcn/1 -> p_BP_out/1
  Integrator/1 -> Abs/1  "v"

== system Simulation/Subsystem10/Wagon model4 ==
  p_BP : Inport
  Abs : Abs
  Constant : Constant  Value=m
  Divide : Product  Inputs=*/
  Gain : Gain  Gain=-1/(RBD-VBD)
  Gain1 : Gain  Gain=Fb
  Gravity : Gain  Gain=9.81
  Integrator : Integrator  InitialCondition=v0
  Product : Product
  Rate Limiter : RateLimiter  RisingSlewLimit=1/tf  FallingSlewLimit=-1/tl  SampleTimeMode=inherited
  Saturation : Saturate  UpperLimit=1  LowerLimit=0
  Strahl formula : Polyval  Coefs=Pres
  Sum1 : Sum  Inputs=|+-
  Transfer Fcn : TransferFcn  Numerator=BPnum  Denominator=BPden
  Transport Delay : TransportDelay  DelayTime=l/c  InitialOutput=p0
  Fres : Outport
  p_BP_out : Outport  Port=2
  wires:
  Sum1/1 -> Fres/1, Divide/1  "Fres"
  Strahl formula/1 -> Gravity/1
  Abs/1 -> Strahl formula/1
  Gravity/1 -> Product/2
  Product/1 -> Sum1/2  "Fw"
  Integrator/1 -> Abs/1  "v"
  Constant/1 -> Product/1, Divide/2
  Divide/1 -> Integrator/1  "a"
  p_BP/1 -> Gain/1, Transport Delay/1
  Gain/1 -> Saturation/1
  Gain1/1 -> Sum1/1
  Saturation/1 -> Rate Limiter/1
  Rate Limiter/1 -> Gain1/1
  Transfer Fcn/1 -> p_BP_out/1
  Transport Delay/1 -> Transfer Fcn/1

== system Simulation/Subsystem11/Wagon model ==
  p_BP : Inport
  Abs : Abs
  Constant : Constant  Value=m
  Divide : Product  Inputs=*/
  Gain : Gain  Gain=-1/(RBD-VBD)
  Gain1 : Gain  Gain=Fb
  Gravity : Gain  Gain=9.81
  Integrator : Integrator  InitialCondition=v0
  Product : Product
  Rate Limiter : RateLimiter  RisingSlewLimit=1/tf  FallingSlewLimit=-1/tl  SampleTimeMode=inherited
  Saturation : Saturate  UpperLimit=1  LowerLimit=0
  Strahl formula : Polyval  Coefs=Pres
  Sum1 : Sum  Inputs=|+-
  Transfer Fcn : TransferFcn  Numerator=BPnum  Denominator=BPden
  Transport Delay : TransportDelay  DelayTime=l/c  InitialOutput=p0
  Fres : Outport
  p_BP_out : Outport  Port=2
  wires:
  Sum1/1 -> Fres/1, Divide/1  "Fres"
  Strahl formula/1 -> Gravity/1
  Abs/1 -> Strahl formula/1
  Gravity/1 -> Product/2
  Product/1 -> Sum1/2  "Fw"
  Integrator/1 -> Abs/1  "v"
  Constant/1 -> Product/1, Divide/2
  Divide/1 -> Integrator/1  "a"
  p_BP/1 -> Gain/1, Transport Delay/1
  Gain/1 -> Saturation/1
  Gain1/1 -> Sum1/1
  Saturation/1 -> Rate Limiter/1
  Rate Limiter/1 -> Gain1/1
  Transfer Fcn/1 -> p_BP_out/1
  Transport Delay/1 -> Transfer Fcn/1

== system Simulation/Subsystem11/Wagon model1 ==
  p_BP : Inport
  Abs : Abs
  Constant : Constant  Value=m
  Divide : Product  Inputs=*/
  Gain : Gain  Gain=-1/(RBD-VBD)
  Gain1 : Gain  Gain=Fb
  Gravity : Gain  Gain=9.81
  Integrator : Integrator  InitialCondition=v0
  Product : Product
  Rate Limiter : RateLimiter  RisingSlewLimit=1/tf  FallingSlewLimit=-1/tl  SampleTimeMode=inherited
  Saturation : Saturate  UpperLimit=1  LowerLimit=0
  Strahl formula : Polyval  Coefs=Pres
  Sum1 : Sum  Inputs=|+-
  Transfer Fcn : TransferFcn  Numerator=BPnum  Denominator=BPden
  Transport Delay : TransportDelay  DelayTime=l/c  InitialOutput=p0
  Fres : Outport
  p_BP_out : Outport  Port=2
  wires:
  Sum1/1 -> Fres/1, Divide/1  "Fres"
  Strahl formula/1 -> Gravity/1
  Abs/1 -> Strahl formula/1
  Gravity/1 -> Product/2
  Product/1 -> Sum1/2  "Fw"
  Integrator/1 -> Abs/1  "v"
  Constant/1 -> Product/1, Divide/2
  Divide/1 -> Integrator/1  "a"
  p_BP/1 -> Gain/1, Transport Delay/1
  Gain/1 -> Saturation/1
  Gain1/1 -> Sum1/1
  Saturation/1 -> Rate Limiter/1
  Rate Limiter/1 -> Gain1/1
  Transport Delay/1 -> Transfer Fcn/1
  Transfer Fcn/1 -> p_BP_out/1

== system Simulation/Subsystem11/Wagon model2 ==
  p_BP : Inport
  Abs : Abs
  Constant : Constant  Value=m
  Divide : Product  Inputs=*/
  Gain : Gain  Gain=-1/(RBD-VBD)
  Gain1 : Gain  Gain=Fb
  Gravity : Gain  Gain=9.81
  Integrator : Integrator  InitialCondition=v0
  Product : Product
  Rate Limiter : RateLimiter  RisingSlewLimit=1/tf  FallingSlewLimit=-1/tl  SampleTimeMode=inherited
  Saturation : Saturate  UpperLimit=1  LowerLimit=0
  Strahl formula : Polyval  Coefs=Pres
  Sum1 : Sum  Inputs=|+-
  Transfer Fcn : TransferFcn  Numerator=BPnum  Denominator=BPden
  Transport Delay : TransportDelay  DelayTime=l/c  InitialOutput=p0
  Fres : Outport
  p_BP_out : Outport  Port=2
  wires:
  Sum1/1 -> Fres/1, Divide/1  "Fres"
  Strahl formula/1 -> Gravity/1
  Abs/1 -> Strahl formula/1
  Gravity/1 -> Product/2
  Product/1 -> Sum1/2  "Fw"
  Constant/1 -> Product/1, Divide/2
  Divide/1 -> Integrator/1  "a"
  p_BP/1 -> Gain/1, Transport Delay/1
  Gain/1 -> Saturation/1
  Gain1/1 -> Sum1/1
  Saturation/1 -> Rate Limiter/1
  Rate Limiter/1 -> Gain1/1
  Transport Delay/1 -> Transfer Fcn/1
  Transfer Fcn/1 -> p_BP_out/1
  Integrator/1 -> Abs/1  "v"

== system Simulation/Subsystem11/Wagon model3 ==
  p_BP : Inport
  Abs : Abs
  Constant : Constant  Value=m
  Divide : Product  Inputs=*/
  Gain : Gain  Gain=-1/(RBD-VBD)
  Gain1 : Gain  Gain=Fb
  Gravity : Gain  Gain=9.81
  Integrator : Integrator  InitialCondition=v0
  Product : Product
  Rate Limiter : RateLimiter  RisingSlewLimit=1/tf  FallingSlewLimit=-1/tl  SampleTimeMode=inherited
  Saturation : Saturate  UpperLimit=1  LowerLimit=0
  Strahl formula : Polyval  Coefs=Pres
  Sum1 : Sum  Inputs=|+-
  Transfer Fcn : TransferFcn  Numerator=BPnum  Denominator=BPden
  Transport Delay : TransportDelay  DelayTime=l/c  InitialOutput=p0
  Fres : Outport
  p_BP_out : Outport  Port=2
  wires:
  Sum1/1 -> Fres/1, Divide/1  "Fres"
  Strahl formula/1 -> Gravity/1
  Abs/1 -> Strahl formula/1
  Gravity/1 -> Product/2
  Product/1 -> Sum1/2  "Fw"
  Constant/1 -> Product/1, Divide/2
  Divide/1 -> Integrator/1  "a"
  p_BP/1 -> Gain/1, Transport Delay/1
  Gain/1 -> Saturation/1
  Gain1/1 -> Sum1/1
  Saturation/1 -> Rate Limiter/1
  Rate Limiter/1 -> Gain1/1
  Transport Delay/1 -> Transfer Fcn/1
  Transfer Fcn/1 -> p_BP_out/1
  Integrator/1 -> Abs/1  "v"

== system Simulation/Subsystem11/Wagon model4 ==
  p_BP : Inport
  Abs : Abs
  Constant : Constant  Value=m
  Divide : Product  Inputs=*/
  Gain : Gain  Gain=-1/(RBD-VBD)
  Gain1 : Gain  Gain=Fb
  Gravity : Gain  Gain=9.81
  Integrator : Integrator  InitialCondition=v0
  Product : Product
  Rate Limiter : RateLimiter  RisingSlewLimit=1/tf  FallingSlewLimit=-1/tl  SampleTimeMode=inherited
  Saturation : Saturate  UpperLimit=1  LowerLimit=0
  Strahl formula : Polyval  Coefs=Pres
  Sum1 : Sum  Inputs=|+-
  Transfer Fcn : TransferFcn  Numerator=BPnum  Denominator=BPden
  Transport Delay : TransportDelay  DelayTime=l/c  InitialOutput=p0
  Fres : Outport
  p_BP_out : Outport  Port=2
  wires:
  Sum1/1 -> Fres/1, Divide/1  "Fres"
  Strahl formula/1 -> Gravity/1
  Abs/1 -> Strahl formula/1
  Gravity/1 -> Product/2
  Product/1 -> Sum1/2  "Fw"
  Integrator/1 -> Abs/1  "v"
  Constant/1 -> Product/1, Divide/2
  Divide/1 -> Integrator/1  "a"
  p_BP/1 -> Gain/1, Transport Delay/1
  Gain/1 -> Saturation/1
  Gain1/1 -> Sum1/1
  Saturation/1 -> Rate Limiter/1
  Rate Limiter/1 -> Gain1/1
  Transfer Fcn/1 -> p_BP_out/1
  Transport Delay/1 -> Transfer Fcn/1

== system Simulation/Subsystem12/Wagon model ==
  p_BP : Inport
  Abs : Abs
  Constant : Constant  Value=m
  Divide : Product  Inputs=*/
  Gain : Gain  Gain=-1/(RBD-VBD)
  Gain1 : Gain  Gain=Fb
  Gravity : Gain  Gain=9.81
  Integrator : Integrator  InitialCondition=v0
  Product : Product
  Rate Limiter : RateLimiter  RisingSlewLimit=1/tf  FallingSlewLimit=-1/tl  SampleTimeMode=inherited
  Saturation : Saturate  UpperLimit=1  LowerLimit=0
  Strahl formula : Polyval  Coefs=Pres
  Sum1 : Sum  Inputs=|+-
  Transfer Fcn : TransferFcn  Numerator=BPnum  Denominator=BPden
  Transport Delay : TransportDelay  DelayTime=l/c  InitialOutput=p0
  Fres : Outport
  p_BP_out : Outport  Port=2
  wires:
  Sum1/1 -> Fres/1, Divide/1  "Fres"
  Strahl formula/1 -> Gravity/1
  Abs/1 -> Strahl formula/1
  Gravity/1 -> Product/2
  Product/1 -> Sum1/2  "Fw"
  Integrator/1 -> Abs/1  "v"
  Constant/1 -> Product/1, Divide/2
  Divide/1 -> Integrator/1  "a"
  p_BP/1 -> Gain/1, Transport Delay/1
  Gain/1 -> Saturation/1
  Gain1/1 -> Sum1/1
  Saturation/1 -> Rate Limiter/1
  Rate Limiter/1 -> Gain1/1
  Transfer Fcn/1 -> p_BP_out/1
  Transport Delay/1 -> Transfer Fcn/1

== system Simulation/Subsystem12/Wagon model1 ==
  p_BP : Inport
  Abs : Abs
  Constant : Constant  Value=m
  Divide : Product  Inputs=*/
  Gain : Gain  Gain=-1/(RBD-VBD)
  Gain1 : Gain  Gain=Fb
  Gravity : Gain  Gain=9.81
  Integrator : Integrator  InitialCondition=v0
  Product : Product
  Rate Limiter : RateLimiter  RisingSlewLimit=1/tf  FallingSlewLimit=-1/tl  SampleTimeMode=inherited
  Saturation : Saturate  UpperLimit=1  LowerLimit=0
  Strahl formula : Polyval  Coefs=Pres
  Sum1 : Sum  Inputs=|+-
  Transfer Fcn : TransferFcn  Numerator=BPnum  Denominator=BPden
  Transport Delay : TransportDelay  DelayTime=l/c  InitialOutput=p0
  Fres : Outport
  p_BP_out : Outport  Port=2
  wires:
  Sum1/1 -> Fres/1, Divide/1  "Fres"
  Strahl formula/1 -> Gravity/1
  Abs/1 -> Strahl formula/1
  Gravity/1 -> Product/2
  Product/1 -> Sum1/2  "Fw"
  Integrator/1 -> Abs/1  "v"
  Constant/1 -> Product/1, Divide/2
  Divide/1 -> Integrator/1  "a"
  p_BP/1 -> Gain/1, Transport Delay/1
  Gain/1 -> Saturation/1
  Gain1/1 -> Sum1/1
  Saturation/1 -> Rate Limiter/1
  Rate Limiter/1 -> Gain1/1
  Transport Delay/1 -> Transfer Fcn/1
  Transfer Fcn/1 -> p_BP_out/1

== system Simulation/Subsystem12/Wagon model2 ==
  p_BP : Inport
  Abs : Abs
  Constant : Constant  Value=m
  Divide : Product  Inputs=*/
  Gain : Gain  Gain=-1/(RBD-VBD)
  Gain1 : Gain  Gain=Fb
  Gravity : Gain  Gain=9.81
  Integrator : Integrator  InitialCondition=v0
  Product : Product
  Rate Limiter : RateLimiter  RisingSlewLimit=1/tf  FallingSlewLimit=-1/tl  SampleTimeMode=inherited
  Saturation : Saturate  UpperLimit=1  LowerLimit=0
  Strahl formula : Polyval  Coefs=Pres
  Sum1 : Sum  Inputs=|+-
  Transfer Fcn : TransferFcn  Numerator=BPnum  Denominator=BPden
  Transport Delay : TransportDelay  DelayTime=l/c  InitialOutput=p0
  Fres : Outport
  p_BP_out : Outport  Port=2
  wires:
  Sum1/1 -> Fres/1, Divide/1  "Fres"
  Strahl formula/1 -> Gravity/1
  Abs/1 -> Strahl formula/1
  Gravity/1 -> Product/2
  Product/1 -> Sum1/2  "Fw"
  Constant/1 -> Product/1, Divide/2
  Divide/1 -> Integrator/1  "a"
  p_BP/1 -> Gain/1, Transport Delay/1
  Gain/1 -> Saturation/1
  Gain1/1 -> Sum1/1
  Saturation/1 -> Rate Limiter/1
  Rate Limiter/1 -> Gain1/1
  Transport Delay/1 -> Transfer Fcn/1
  Transfer Fcn/1 -> p_BP_out/1
  Integrator/1 -> Abs/1  "v"

== system Simulation/Subsystem12/Wagon model3 ==
  p_BP : Inport
  Abs : Abs
  Constant : Constant  Value=m
  Divide : Product  Inputs=*/
  Gain : Gain  Gain=-1/(RBD-VBD)
  Gain1 : Gain  Gain=Fb
  Gravity : Gain  Gain=9.81
  Integrator : Integrator  InitialCondition=v0
  Product : Product
  Rate Limiter : RateLimiter  RisingSlewLimit=1/tf  FallingSlewLimit=-1/tl  SampleTimeMode=inherited
  Saturation : Saturate  UpperLimit=1  LowerLimit=0
  Strahl formula : Polyval  Coefs=Pres
  Sum1 : Sum  Inputs=|+-
  Transfer Fcn : TransferFcn  Numerator=BPnum  Denominator=BPden
  Transport Delay : TransportDelay  DelayTime=l/c  InitialOutput=p0
  Fres : Outport
  p_BP_out : Outport  Port=2
  wires:
  Sum1/1 -> Fres/1, Divide/1  "Fres"
  Strahl formula/1 -> Gravity/1
  Abs/1 -> Strahl formula/1
  Gravity/1 -> Product/2
  Product/1 -> Sum1/2  "Fw"
  Constant/1 -> Product/1, Divide/2
  Divide/1 -> Integrator/1  "a"
  p_BP/1 -> Gain/1, Transport Delay/1
  Gain/1 -> Saturation/1
  Gain1/1 -> Sum1/1
  Saturation/1 -> Rate Limiter/1
  Rate Limiter/1 -> Gain1/1
  Transport Delay/1 -> Transfer Fcn/1
  Transfer Fcn/1 -> p_BP_out/1
  Integrator/1 -> Abs/1  "v"

== system Simulation/Subsystem12/Wagon model4 ==
  p_BP : Inport
  Abs : Abs
  Constant : Constant  Value=m
  Divide : Product  Inputs=*/
  Gain : Gain  Gain=-1/(RBD-VBD)
  Gain1 : Gain  Gain=Fb
  Gravity : Gain  Gain=9.81
  Integrator : Integrator  InitialCondition=v0
  Product : Product
  Rate Limiter : RateLimiter  RisingSlewLimit=1/tf  FallingSlewLimit=-1/tl  SampleTimeMode=inherited
  Saturation : Saturate  UpperLimit=1  LowerLimit=0
  Strahl formula : Polyval  Coefs=Pres
  Sum1 : Sum  Inputs=|+-
  Transfer Fcn : TransferFcn  Numerator=BPnum  Denominator=BPden
  Transport Delay : TransportDelay  DelayTime=l/c  InitialOutput=p0
  Fres : Outport
  p_BP_out : Outport  Port=2
  wires:
  Sum1/1 -> Fres/1, Divide/1  "Fres"
  Strahl formula/1 -> Gravity/1
  Abs/1 -> Strahl formula/1
  Gravity/1 -> Product/2
  Product/1 -> Sum1/2  "Fw"
  Integrator/1 -> Abs/1  "v"
  Constant/1 -> Product/1, Divide/2
  Divide/1 -> Integrator/1  "a"
  p_BP/1 -> Gain/1, Transport Delay/1
  Gain/1 -> Saturation/1
  Gain1/1 -> Sum1/1
  Saturation/1 -> Rate Limiter/1
  Rate Limiter/1 -> Gain1/1
  Transfer Fcn/1 -> p_BP_out/1
  Transport Delay/1 -> Transfer Fcn/1

== system Simulation/Subsystem13/Wagon model ==
  p_BP : Inport
  Abs : Abs
  Constant : Constant  Value=m
  Divide : Product  Inputs=*/
  Gain : Gain  Gain=-1/(RBD-VBD)
  Gain1 : Gain  Gain=Fb
  Gravity : Gain  Gain=9.81
  Integrator : Integrator  InitialCondition=v0
  Product : Product
  Rate Limiter : RateLimiter  RisingSlewLimit=1/tf  FallingSlewLimit=-1/tl  SampleTimeMode=inherited
  Saturation : Saturate  UpperLimit=1  LowerLimit=0
  Strahl formula : Polyval  Coefs=Pres
  Sum1 : Sum  Inputs=|+-
  Transfer Fcn : TransferFcn  Numerator=BPnum  Denominator=BPden
  Transport Delay : TransportDelay  DelayTime=l/c  InitialOutput=p0
  Fres : Outport
  p_BP_out : Outport  Port=2
  wires:
  Sum1/1 -> Fres/1, Divide/1  "Fres"
  Strahl formula/1 -> Gravity/1
  Abs/1 -> Strahl formula/1
  Gravity/1 -> Product/2
  Product/1 -> Sum1/2  "Fw"
  Integrator/1 -> Abs/1  "v"
  Constant/1 -> Product/1, Divide/2
  Divide/1 -> Integrator/1  "a"
  p_BP/1 -> Gain/1, Transport Delay/1
  Gain/1 -> Saturation/1
  Gain1/1 -> Sum1/1
  Saturation/1 -> Rate Limiter/1
  Rate Limiter/1 -> Gain1/1
  Transfer Fcn/1 -> p_BP_out/1
  Transport Delay/1 -> Transfer Fcn/1

== system Simulation/Subsystem13/Wagon model1 ==
  p_BP : Inport
  Abs : Abs
  Constant : Constant  Value=m
  Divide : Product  Inputs=*/
  Gain : Gain  Gain=-1/(RBD-VBD)
  Gain1 : Gain  Gain=Fb
  Gravity : Gain  Gain=9.81
  Integrator : Integrator  InitialCondition=v0
  Product : Product
  Rate Limiter : RateLimiter  RisingSlewLimit=1/tf  FallingSlewLimit=-1/tl  SampleTimeMode=inherited
  Saturation : Saturate  UpperLimit=1  LowerLimit=0
  Strahl formula : Polyval  Coefs=Pres
  Sum1 : Sum  Inputs=|+-
  Transfer Fcn : TransferFcn  Numerator=BPnum  Denominator=BPden
  Transport Delay : TransportDelay  DelayTime=l/c  InitialOutput=p0
  Fres : Outport
  p_BP_out : Outport  Port=2
  wires:
  Sum1/1 -> Fres/1, Divide/1  "Fres"
  Strahl formula/1 -> Gravity/1
  Abs/1 -> Strahl formula/1
  Gravity/1 -> Product/2
  Product/1 -> Sum1/2  "Fw"
  Integrator/1 -> Abs/1  "v"
  Constant/1 -> Product/1, Divide/2
  Divide/1 -> Integrator/1  "a"
  p_BP/1 -> Gain/1, Transport Delay/1
  Gain/1 -> Saturation/1
  Gain1/1 -> Sum1/1
  Saturation/1 -> Rate Limiter/1
  Rate Limiter/1 -> Gain1/1
  Transport Delay/1 -> Transfer Fcn/1
  Transfer Fcn/1 -> p_BP_out/1
